simulink model "BlockDiagram"  (R2021a)
settings: Solver=VariableStepAuto  StartTime=0.0  StopTime=10.0  RelTol=1e-3
undefined symbols (not defined in the file): B, J, K, L, R
settings Model: Creator=Fady  LastModifiedBy=Fady

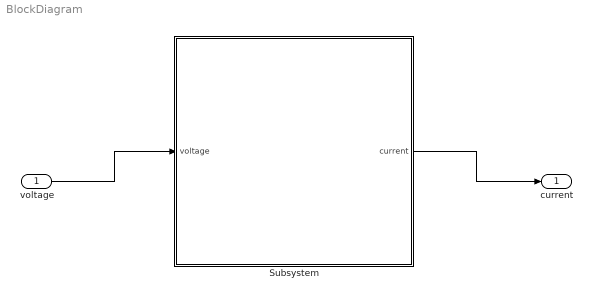
== system BlockDiagram ==
  voltage : Inport
  Subsystem : Subsystem
  current : Outport
  wires:
  voltage/1 -> Subsystem/1(voltage)
  Subsystem/1(current) -> current/1

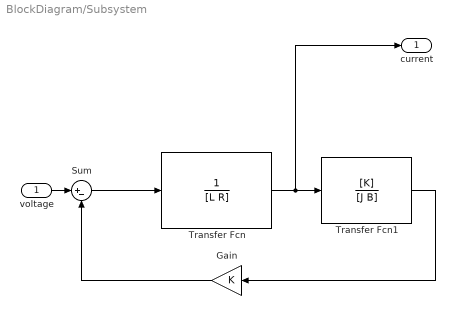
== system BlockDiagram/Subsystem ==
  voltage : Inport
  Gain : Gain  Gain=K
  Sum : Sum  Inputs=|+-
  Transfer Fcn : TransferFcn  Denominator=[L R]
  Transfer Fcn1 : TransferFcn  Numerator=[K]  Denominator=[J B]
  current : Outport
  wires:
  Transfer Fcn1/1 -> Gain/1
  Sum/1 -> Transfer Fcn/1
  Gain/1 -> Sum/2
  voltage/1 -> Sum/1
  Transfer Fcn/1 -> current/1, Transfer Fcn1/1
